simulink model "Par_model_sim_CHB5"  (R2023b)
settings: Solver=FixedStepAuto  StartTime=0.0  StopTime=5  FixedStep=1e-6  RelTol=1e-3
InitFcn:
  | sysinit
values from neighbouring files (symbols this model uses):
  C = 0.0234    [sysinit.m]
  f_out = frequency_out_start : frequency_out_interval : frequency_out_end    [simout_chb_par.m]    (also in simout_chbjt_par.m = frequency_modulate_start : frequency_modulate_interval : fre)
  f_switch = 250    [sysinit.m]
  fn = 50    [sysinit.m]
  L = 0.002    [sysinit.m]
  L_ori = 0.02    [sysinit.m]
  L_sec = 0.06    [sysinit.m]
  m_par = modulate_radio_start : modulate_radio_interval : modulate_radio_end    [simout_chb_par.m]
  P0 = 8e6    (= 8000000)    [sysinit.m]
  R = 1.5    [sysinit.m]
  Source_Amp = 10000    [sysinit.m]
  st = 1e-6    (= 1e-06)    [sysinit.m]
  Td = 15e-7    (= 1.5e-06)    [sysinit.m]
  Ul_in = 1900    [sysinit.m]
undefined symbols (not defined in the file or in its folder): D1, Delta
libraries: spsSeriesRLCBranchLib x63, spsDiodeLib x30, simulink x24, spsIGBTLib x24, spsCurrentMeasurementLib x10, spsThreePhaseVIMeasurementLib x7, spsOnDelayLib x6, spsUniversalBridgeLib x6, spsVoltageMeasurementLib x3, spsThreePhaseTransformerThreeWindingsLib x3, spsThreePhaseProgrammableVoltageSourceLib x1, spsGroundLib x1
(part 2 of 2)

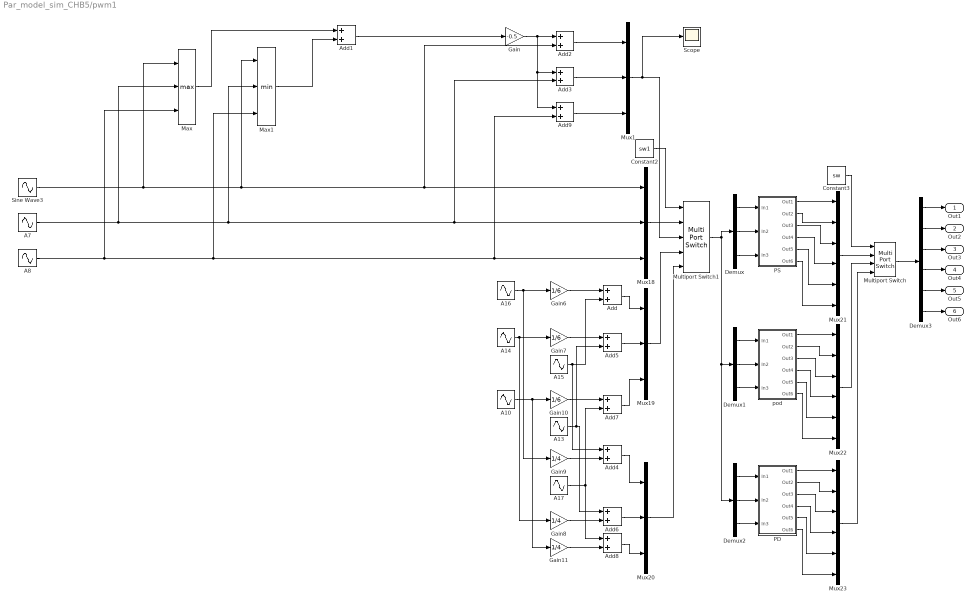
== system Par_model_sim_CHB5/pwm1 ==
  A10 : Sin  Amplitude=m*1000  Frequency=2*pi*f*3  Phase=pi+2*pi/3  SampleTime=0
  A13 : Sin  Amplitude=m*1000  Frequency=2*pi*f  Phase=pi-2*pi/3  SampleTime=0
  A14 : Sin  Amplitude=m*1000  Frequency=2*pi*f*3  Phase=pi-2*pi/3  SampleTime=0
  A15 : Sin  Amplitude=m*1000  Frequency=2*pi*f  Phase=pi  SampleTime=0
  A16 : Sin  Amplitude=m*1000  Frequency=2*pi*f*3  Phase=pi  SampleTime=0
  A17 : Sin  Amplitude=m*1000  Frequency=2*pi*f  Phase=pi+2*pi/3  SampleTime=0
  A7 : Sin  Amplitude=m*1000  Frequency=2*pi*f  Phase=-2*pi/3  SampleTime=0
  A8 : Sin  Amplitude=m*1000  Frequency=2*pi*f  Phase=2*pi/3  SampleTime=0
  Add{,1..9} (10 alike) : Sum
  Constant2 : Constant  Value=sw1
  Constant3 : Constant  Value=sw
  Demux : Demux  Outputs=3
  Demux1 : Demux  Outputs=3
  Demux2 : Demux  Outputs=3
  Demux3 : Demux  Outputs=6
  Gain : Gain  Gain=-0.5
  Gain10 : Gain  Gain=1/6
  Gain11 : Gain  Gain=1/4
  Gain6 : Gain  Gain=1/6
  Gain7 : Gain  Gain=1/6
  Gain8 : Gain  Gain=1/4
  Gain9 : Gain  Gain=1/4
  Max : MinMax  Function=max  Inputs=3
  Max1 : MinMax  Inputs=3
  Multiport Switch : MultiPortSwitch  SaturateOnIntegerOverflow=off  InputSameDT=off
  Multiport Switch1 : MultiPortSwitch  Inputs=4  SaturateOnIntegerOverflow=off  InputSameDT=off
  Mux{1,18..20} (4 alike) : Mux  Inputs=3
  Mux21 : Mux  Inputs=6
  Mux22 : Mux  Inputs=6
  Mux23 : Mux  Inputs=6
  PD : Subsystem
  PS : Subsystem
  Scope : Scope
  Sine Wave3 : Sin  Amplitude=m*1000  Frequency=2*pi*f  SampleTime=0
  pod : Subsystem
  Out1 : Outport
  Out2 : Outport  Port=2
  Out3 : Outport  Port=3
  Out4 : Outport  Port=4
  Out5 : Outport  Port=5
  Out6 : Outport  Port=6
  wires:
  Gain8/1 -> Add6/2
  Demux3/2 -> Out2/1
  Demux1/1 -> pod/1(In1)
  Mux19/1 -> Multiport Switch1/4
  Demux3/6 -> Out6/1
  A10/1 -> Gain11/1, Gain10/1
  PD/1(Out1) -> Mux23/1
  PD/3(Out3) -> Mux23/3
  PD/2(Out2) -> Mux23/2
  Demux3/5 -> Out5/1
  PD/4(Out4) -> Mux23/4
  A13/1 -> Add5/2, Add6/1
  Demux2/1 -> PD/1(In1)
  Demux2/3 -> PD/3(In3)
  PD/5(Out5) -> Mux23/5
  PD/6(Out6) -> Mux23/6
  Add8/1 -> Mux20/3
  Add7/1 -> Mux19/3
  Add5/1 -> Mux19/2
  Add6/1 -> Mux20/2
  Constant2/1 -> Multiport Switch1/1
  PS/3(Out3) -> Mux21/3
  PS/4(Out4) -> Mux21/4
  PS/5(Out5) -> Mux21/5
  PS/2(Out2) -> Mux21/2
  Constant3/1 -> Multiport Switch/1
  Mux20/1 -> Multiport Switch1/5
  Gain10/1 -> Add7/1
  Gain7/1 -> Add5/1
  Mux21/1 -> Multiport Switch/2
  A8/1 -> Max/3, Max1/3, Add9/2, Mux18/3
  Gain9/1 -> Add4/2
  Gain6/1 -> Add/1
  Gain11/1 -> Add8/2
  Demux1/3 -> pod/3(In3)
  Demux1/2 -> pod/2(In2)
  Demux/3 -> PS/3(In3)
  Demux3/3 -> Out3/1
  Sine Wave3/1 -> Max/1, Max1/1, Add2/2, Mux18/1
  pod/4(Out4) -> Mux22/4
  pod/1(Out1) -> Mux22/1
  pod/3(Out3) -> Mux22/3
  pod/2(Out2) -> Mux22/2
  Demux3/4 -> Out4/1
  Multiport Switch/1 -> Demux3/1
  Demux2/2 -> PD/2(In2)
  Demux/1 -> PS/1(In1)
  Demux/2 -> PS/2(In2)
  pod/6(Out6) -> Mux22/6
  pod/5(Out5) -> Mux22/5
  PS/6(Out6) -> Mux21/6
  Demux3/1 -> Out1/1
  PS/1(Out1) -> Mux21/1
  Add/1 -> Mux19/1
  Add4/1 -> Mux20/1
  Multiport Switch1/1 -> Demux/1, Demux1/1, Demux2/1
  Mux18/1 -> Multiport Switch1/2
  Mux22/1 -> Multiport Switch/3
  Mux23/1 -> Multiport Switch/4
  A17/1 -> Add8/1, Add7/2
  A16/1 -> Gain9/1, Gain6/1
  A15/1 -> Add4/1, Add/2
  A14/1 -> Gain7/1, Gain8/1
  Max/1 -> Add1/1
  Max1/1 -> Add1/2
  Add1/1 -> Gain/1
  Gain/1 -> Add9/1, Add3/1, Add2/1
  Add9/1 -> Mux1/3
  Add3/1 -> Mux1/2
  Add2/1 -> Mux1/1
  A7/1 -> Max/2, Max1/2, Add3/2, Mux18/2
  Mux1/1 -> Scope/1, Multiport Switch1/3

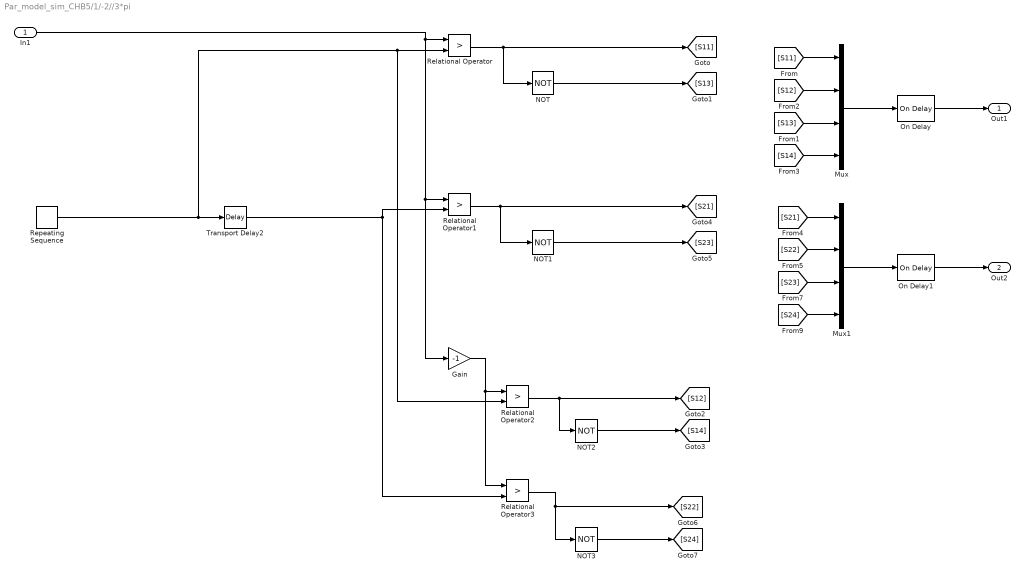
== system Par_model_sim_CHB5/1/-2//3*pi ==
  In1 : Inport
  Gain : Gain  Gain=-1
  Mux : Mux
  Mux1 : Mux
  NOT{,1..3} (4 alike) : Logic  Operator=NOT  AllPortsSameDT=off  OutDataTypeStr=boolean
  On Delay : spsOnDelayLib/On Delay  DelayType=On delay  delay=ttd  ic=0  Ts=0
  On Delay1 : spsOnDelayLib/On Delay  DelayType=On delay  delay=ttd  ic=0  Ts=0
  Relational Operator{,1..3} (4 alike) : RelationalOperator  Operator=>  OutDataTypeStr=boolean  RndMeth=Simplest  InputSameDT=off
  Repeating Sequence : simulink/Sources/Repeating Sequence  rep_seq_t=[0 0.5 1]/f_car  rep_seq_y=[-1 1 -1]*1000
  Transport Delay2 : TransportDelay  DelayTime=tt/f_car  BufferSize=3072
  Out1 : Outport
  Out2 : Outport  Port=2
  wires:
  On Delay1/1 -> Out2/1
  On Delay/1 -> Out1/1
  NOT/1 -> [S13]
  Transport Delay2/1 -> Relational Operator1/2, Relational Operator3/2
  [S14] -> Mux/4
  [S23] -> Mux1/3
  [S12] -> Mux/2
  In1/1 -> Gain/1, Relational Operator1/1, Relational Operator/1
  NOT2/1 -> [S14]
  [S21] -> Mux1/1
  Relational Operator1/1 -> NOT1/1, [S21]
  [S22] -> Mux1/2
  NOT3/1 -> [S24]
  Mux/1 -> On Delay/1
  Repeating Sequence/1 -> Relational Operator2/2, Relational Operator/2, Transport Delay2/1
  [S24] -> Mux1/4
  Gain/1 -> Relational Operator3/1, Relational Operator2/1
  [S13] -> Mux/3
  Relational Operator2/1 -> NOT2/1, [S12]
  [S11] -> Mux/1
  Relational Operator/1 -> NOT/1, [S11]
  NOT1/1 -> [S23]
  Mux1/1 -> On Delay1/1
  Relational Operator3/1 -> [S22], NOT3/1

== system Par_model_sim_CHB5/1/0 ==
  In1 : Inport
  Gain : Gain  Gain=-1
  Mux : Mux
  Mux1 : Mux
  NOT{,1..3} (4 alike) : Logic  Operator=NOT  AllPortsSameDT=off  OutDataTypeStr=boolean
  On Delay1 : spsOnDelayLib/On Delay  DelayType=On delay  delay=ttd  ic=0  Ts=0
  On Delay2 : spsOnDelayLib/On Delay  DelayType=On delay  delay=ttd  ic=0  Ts=0
  Relational Operator{,1..3} (4 alike) : RelationalOperator  Operator=>  OutDataTypeStr=boolean  RndMeth=Simplest  InputSameDT=off
  Repeating Sequence : simulink/Sources/Repeating Sequence  rep_seq_t=[0 0.5 1]/f_car  rep_seq_y=[-1 1 -1]*1000
  Transport Delay2 : TransportDelay  DelayTime=tt/f_car  BufferSize=3072
  Out1 : Outport
  Out2 : Outport  Port=2
  wires:
  On Delay2/1 -> Out1/1
  On Delay1/1 -> Out2/1
  Relational Operator3/1 -> NOT3/1, [S22]
  Mux1/1 -> On Delay1/1
  NOT1/1 -> [S23]
  Relational Operator/1 -> [S11], NOT/1
  [S11] -> Mux/1
  Relational Operator2/1 -> [S12], NOT2/1
  [S13] -> Mux/3
  Gain/1 -> Relational Operator2/1, Relational Operator3/1
  [S24] -> Mux1/4
  Repeating Sequence/1 -> Transport Delay2/1, Relational Operator/2, Relational Operator2/2
  Mux/1 -> On Delay2/1
  NOT3/1 -> [S24]
  [S22] -> Mux1/2
  Relational Operator1/1 -> [S21], NOT1/1
  [S21] -> Mux1/1
  NOT2/1 -> [S14]
  In1/1 -> Relational Operator/1, Relational Operator1/1, Gain/1
  [S12] -> Mux/2
  [S23] -> Mux1/3
  [S14] -> Mux/4
  Transport Delay2/1 -> Relational Operator3/2, Relational Operator1/2
  NOT/1 -> [S13]

== system Par_model_sim_CHB5/1/2//3*pi ==
  In1 : Inport
  Gain : Gain  Gain=-1
  Mux : Mux
  Mux1 : Mux
  NOT{,1..3} (4 alike) : Logic  Operator=NOT  AllPortsSameDT=off  OutDataTypeStr=boolean
  On Delay : spsOnDelayLib/On Delay  DelayType=On delay  delay=ttd  ic=0  Ts=0
  On Delay1 : spsOnDelayLib/On Delay  DelayType=On delay  delay=ttd  ic=0  Ts=0
  Relational Operator{,1..3} (4 alike) : RelationalOperator  Operator=>  OutDataTypeStr=boolean  RndMeth=Simplest  InputSameDT=off
  Repeating Sequence : simulink/Sources/Repeating Sequence  rep_seq_t=[0 0.5 1]/f_car  rep_seq_y=[-1 1 -1]*1000
  Transport Delay2 : TransportDelay  DelayTime=tt/f_car  BufferSize=3072
  Out1 : Outport
  Out2 : Outport  Port=2
  wires:
  On Delay1/1 -> Out2/1
  On Delay/1 -> Out1/1
  Relational Operator3/1 -> NOT3/1, [S22]
  Mux1/1 -> On Delay1/1
  NOT1/1 -> [S23]
  Relational Operator/1 -> [S11], NOT/1
  [S11] -> Mux/1
  Relational Operator2/1 -> [S12], NOT2/1
  [S13] -> Mux/3
  Gain/1 -> Relational Operator2/1, Relational Operator3/1
  [S24] -> Mux1/4
  Repeating Sequence/1 -> Transport Delay2/1, Relational Operator/2, Relational Operator2/2
  Mux/1 -> On Delay/1
  NOT3/1 -> [S24]
  [S22] -> Mux1/2
  Relational Operator1/1 -> [S21], NOT1/1
  [S21] -> Mux1/1
  NOT2/1 -> [S14]
  In1/1 -> Relational Operator/1, Relational Operator1/1, Gain/1
  [S12] -> Mux/2
  [S23] -> Mux1/3
  [S14] -> Mux/4
  Transport Delay2/1 -> Relational Operator3/2, Relational Operator1/2
  NOT/1 -> [S13]

== system Par_model_sim_CHB5/1/Subsystem ==
  In1 : Inport
  In2 : Inport  Port=2
  In3 : Inport  Port=3
  Add{1..3,9} (4 alike) : Sum
  Gain : Gain  Gain=-0.5
  Max : MinMax  Function=max  Inputs=3
  Max1 : MinMax  Inputs=3
  Out1 : Outport
  Out2 : Outport  Port=2
  Out3 : Outport  Port=3
  wires:
  Add3/1 -> Out2/1
  Add2/1 -> Out1/1
  Add9/1 -> Out3/1
  Add1/1 -> Gain/1
  Max1/1 -> Add1/2
  Max/1 -> Add1/1
  Gain/1 -> Add2/1, Add3/1, Add9/1
  In1/1 -> Max/1, Add2/2, Max1/1
  In3/1 -> Max/3, Max1/3, Add9/2
  In2/1 -> Max/2, Max1/2, Add3/2

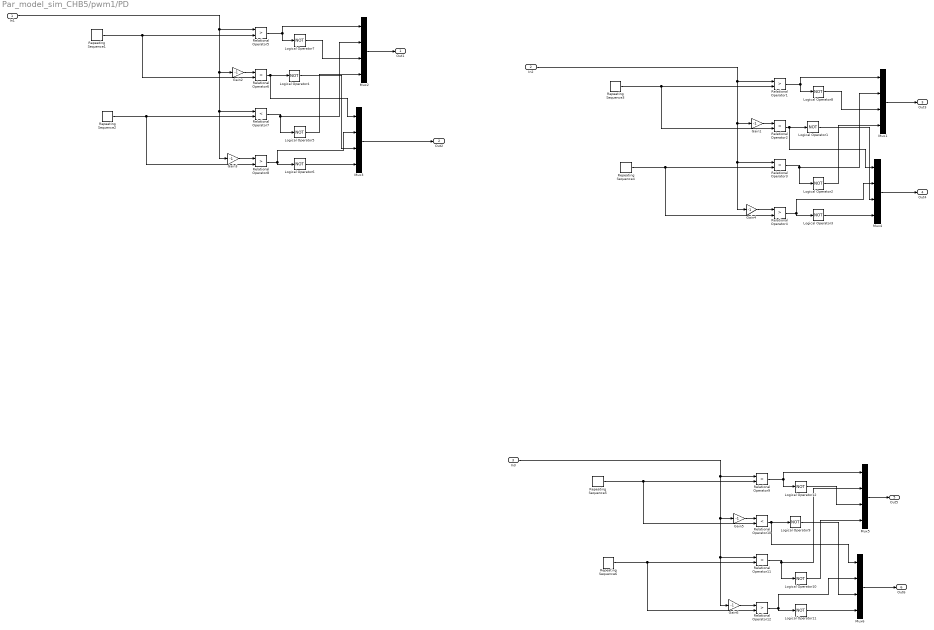
== system Par_model_sim_CHB5/pwm1/PD ==
  In1 : Inport
  In2 : Inport  Port=2
  In3 : Inport  Port=3
  Gain{1..6} (6 alike) : Gain  Gain=-1
  Logical Operator{1..12} (12 alike) : Logic  Operator=NOT  AllPortsSameDT=off  OutDataTypeStr=boolean
  Mux{1..6} (6 alike) : Mux
  Relational Operator{1,4..5,8..9,12} (6 alike) : RelationalOperator  Operator=>  OutDataTypeStr=boolean  RndMeth=Simplest  InputSameDT=off
  Relational Operator{2..3,6..7,10..11} (6 alike) : RelationalOperator  Operator=<  OutDataTypeStr=boolean  RndMeth=Simplest  InputSameDT=off
  Repeating Sequence1 : simulink/Sources/Repeating Sequence  rep_seq_t=[0 0.5 1]/f_carrier  rep_seq_y=[0 1 0]*1000
  Repeating Sequence2 : simulink/Sources/Repeating Sequence  rep_seq_t=[0 0.5 1]/f_carrier  rep_seq_y=[-1 0 -1]*1000
  Repeating Sequence3 : simulink/Sources/Repeating Sequence  rep_seq_t=[0 0.5 1]/f_carrier  rep_seq_y=[0 1 0]*1000
  Repeating Sequence4 : simulink/Sources/Repeating Sequence  rep_seq_t=[0 0.5 1]/f_carrier  rep_seq_y=[-1 0 -1]*1000
  Repeating Sequence5 : simulink/Sources/Repeating Sequence  rep_seq_t=[0 0.5 1]/f_carrier  rep_seq_y=[0 1 0]*1000
  Repeating Sequence6 : simulink/Sources/Repeating Sequence  rep_seq_t=[0 0.5 1]/f_carrier  rep_seq_y=[-1 0 -1]*1000
  Out1 : Outport
  Out2 : Outport  Port=2
  Out3 : Outport  Port=3
  Out4 : Outport  Port=4
  Out5 : Outport  Port=5
  Out6 : Outport  Port=6
  wires:
  Logical Operator4/1 -> Mux3/3
  In1/1 -> Gain3/1, Relational Operator7/1, Gain2/1, Relational Operator5/1
  Relational Operator5/1 -> Logical Operator7/1, Mux2/1
  Gain2/1 -> Relational Operator6/1
  Repeating Sequence1/1 -> Relational Operator6/2, Relational Operator5/2
  Logical Operator7/1 -> Mux2/3
  Logical Operator6/1 -> Mux3/4
  Relational Operator6/1 -> Mux3/1, Logical Operator4/1
  Repeating Sequence2/1 -> Relational Operator8/2, Relational Operator7/2
  Mux3/1 -> Out2/1
  Relational Operator7/1 -> Mux2/2, Logical Operator5/1
  Logical Operator5/1 -> Mux2/4
  Relational Operator8/1 -> Mux3/2, Logical Operator6/1
  Gain3/1 -> Relational Operator8/1
  Mux2/1 -> Out1/1
  Logical Operator1/1 -> Mux4/3
  In2/1 -> Gain4/1, Relational Operator3/1, Gain1/1, Relational Operator1/1
  Relational Operator1/1 -> Logical Operator8/1, Mux1/1
  Gain1/1 -> Relational Operator2/1
  Repeating Sequence3/1 -> Relational Operator2/2, Relational Operator1/2
  Logical Operator8/1 -> Mux1/3
  Logical Operator3/1 -> Mux4/4
  Relational Operator2/1 -> Mux4/1, Logical Operator1/1
  Repeating Sequence4/1 -> Relational Operator4/2, Relational Operator3/2
  Relational Operator3/1 -> Mux1/2, Logical Operator2/1
  Logical Operator2/1 -> Mux1/4
  Relational Operator4/1 -> Mux4/2, Logical Operator3/1
  Gain4/1 -> Relational Operator4/1
  Mux4/1 -> Out4/1
  Mux1/1 -> Out3/1
  Logical Operator9/1 -> Mux6/3
  In3/1 -> Gain6/1, Relational Operator11/1, Gain5/1, Relational Operator9/1
  Relational Operator9/1 -> Logical Operator12/1, Mux5/1
  Gain5/1 -> Relational Operator10/1
  Repeating Sequence5/1 -> Relational Operator10/2, Relational Operator9/2
  Logical Operator12/1 -> Mux5/3
  Logical Operator11/1 -> Mux6/4
  Relational Operator10/1 -> Mux6/1, Logical Operator9/1
  Repeating Sequence6/1 -> Relational Operator12/2, Relational Operator11/2
  Mux6/1 -> Out6/1
  Relational Operator11/1 -> Mux5/2, Logical Operator10/1
  Logical Operator10/1 -> Mux5/4
  Relational Operator12/1 -> Mux6/2, Logical Operator11/1
  Gain6/1 -> Relational Operator12/1
  Mux5/1 -> Out5/1

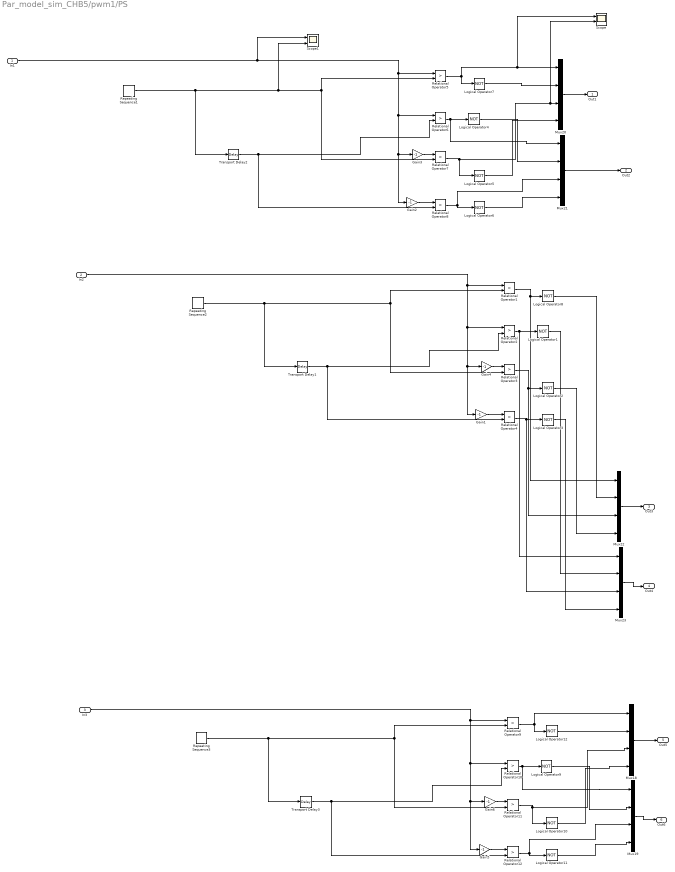
== system Par_model_sim_CHB5/pwm1/PS ==
  In1 : Inport
  In2 : Inport  Port=2
  In3 : Inport  Port=3
  Gain{1..6} (6 alike) : Gain  Gain=-1
  Logical Operator{1..12} (12 alike) : Logic  Operator=NOT  AllPortsSameDT=off  OutDataTypeStr=boolean
  Mux{18..23} (6 alike) : Mux
  Relational Operator{1..12} (12 alike) : RelationalOperator  Operator=>  OutDataTypeStr=boolean  RndMeth=Simplest  InputSameDT=off
  Repeating Sequence1 : simulink/Sources/Repeating Sequence  rep_seq_t=[0 0.5 1]/f_carrier  rep_seq_y=[-1 1 -1]*1000
  Repeating Sequence2 : simulink/Sources/Repeating Sequence  rep_seq_t=[0 0.5 1]/f_carrier  rep_seq_y=[-1 1 -1]*1000
  Repeating Sequence3 : simulink/Sources/Repeating Sequence  rep_seq_t=[0 0.5 1]/f_carrier  rep_seq_y=[-1 1 -1]*1000
  Scope : Scope  NumInputPorts=2
  Scope1 : Scope  NumInputPorts=2
  Transport Delay1 : TransportDelay  DelayTime=0.25*(1/f_carrier)  BufferSize=3072
  Transport Delay2 : TransportDelay  DelayTime=0.25*(1/f_carrier)  BufferSize=3072
  Transport Delay3 : TransportDelay  DelayTime=0.25*(1/f_carrier)  BufferSize=3072
  Out1 : Outport
  Out2 : Outport  Port=2
  Out3 : Outport  Port=3
  Out4 : Outport  Port=4
  Out5 : Outport  Port=5
  Out6 : Outport  Port=6
  wires:
  Mux22/1 -> Out3/1
  Mux18/1 -> Out5/1
  Mux23/1 -> Out4/1
  Mux20/1 -> Out1/1
  Mux19/1 -> Out6/1
  Mux21/1 -> Out2/1
  Logical Operator6/1 -> Mux21/4
  In1/1 -> Scope1/1, Relational Operator6/1, Gain2/1, Gain3/1, Relational Operator5/1
  Logical Operator7/1 -> Mux20/2
  Logical Operator5/1 -> Mux20/4
  Relational Operator7/1 -> Scope/2, Mux20/3, Logical Operator5/1
  Relational Operator8/1 -> Mux21/3, Logical Operator6/1
  Transport Delay2/1 -> Relational Operator8/2, Relational Operator6/2
  Gain3/1 -> Relational Operator7/1
  Relational Operator6/1 -> Mux21/1, Logical Operator4/1
  Logical Operator4/1 -> Mux21/2
  Gain2/1 -> Relational Operator8/1
  Repeating Sequence1/1 -> Transport Delay2/1, Scope1/2, Relational Operator7/2, Relational Operator5/2
  Relational Operator5/1 -> Scope/1, Mux20/1, Logical Operator7/1
  Logical Operator3/1 -> Mux23/4
  In2/1 -> Relational Operator2/1, Gain1/1, Gain4/1, Relational Operator1/1
  Relational Operator3/1 -> Mux22/3, Logical Operator2/1
  Gain4/1 -> Relational Operator3/1
  Transport Delay1/1 -> Relational Operator4/2, Relational Operator2/2
  Relational Operator4/1 -> Mux23/3, Logical Operator3/1
  Logical Operator8/1 -> Mux22/2
  Logical Operator2/1 -> Mux22/4
  Logical Operator1/1 -> Mux23/2
  Relational Operator2/1 -> Mux23/1, Logical Operator1/1
  Gain1/1 -> Relational Operator4/1
  Repeating Sequence2/1 -> Transport Delay1/1, Relational Operator3/2, Relational Operator1/2
  Relational Operator1/1 -> Mux22/1, Logical Operator8/1
  Logical Operator11/1 -> Mux19/4
  In3/1 -> Relational Operator10/1, Gain5/1, Gain6/1, Relational Operator9/1
  Relational Operator11/1 -> Mux18/3, Logical Operator10/1
  Gain6/1 -> Relational Operator11/1
  Transport Delay3/1 -> Relational Operator12/2, Relational Operator10/2
  Relational Operator12/1 -> Mux19/3, Logical Operator11/1
  Logical Operator12/1 -> Mux18/2
  Logical Operator10/1 -> Mux18/4
  Logical Operator9/1 -> Mux19/2
  Relational Operator10/1 -> Mux19/1, Logical Operator9/1
  Gain5/1 -> Relational Operator12/1
  Repeating Sequence3/1 -> Transport Delay3/1, Relational Operator11/2, Relational Operator9/2
  Relational Operator9/1 -> Mux18/1, Logical Operator12/1

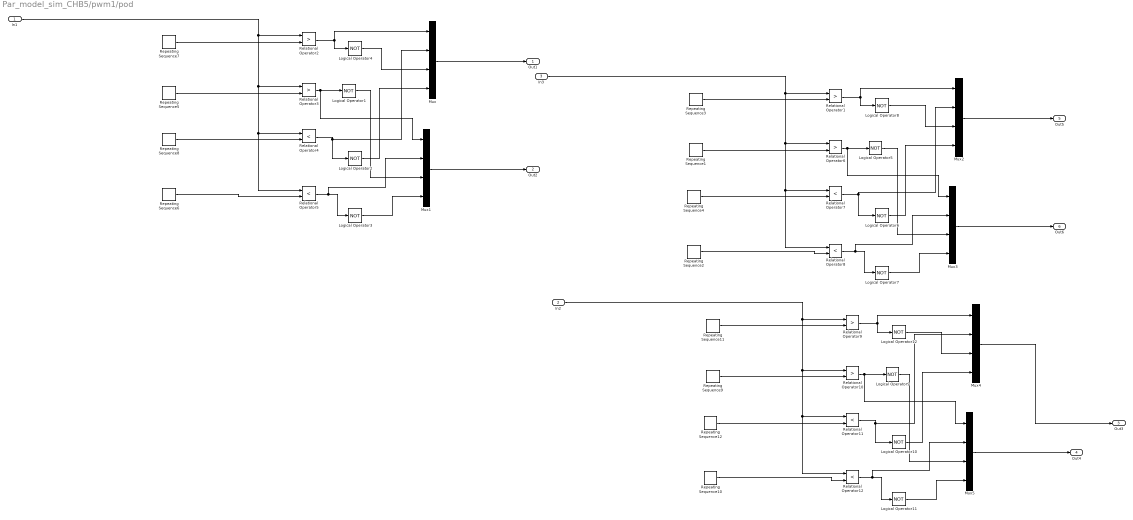
== system Par_model_sim_CHB5/pwm1/pod ==
  In1 : Inport
  In2 : Inport  Port=2
  In3 : Inport  Port=3
  Logical Operator{1..12} (12 alike) : Logic  Operator=NOT  AllPortsSameDT=off  OutDataTypeStr=boolean
  Mux{,1..5} (6 alike) : Mux
  Relational Operator{1..3,6,9..10} (6 alike) : RelationalOperator  Operator=>  OutDataTypeStr=boolean  RndMeth=Simplest  InputSameDT=off
  Relational Operator{4..5,7..8,11..12} (6 alike) : RelationalOperator  Operator=<  OutDataTypeStr=boolean  RndMeth=Simplest  InputSameDT=off
  Repeating Sequence1 : simulink/Sources/Repeating Sequence  rep_seq_t=[0 0.5 1]*(1/f_carrier)  rep_seq_y=[0 1 0]*500
  Repeating Sequence10 : simulink/Sources/Repeating Sequence  rep_seq_t=[0 0.5 1]*(1/f_carrier)  rep_seq_y=[-2 -1 -2]*500
  Repeating Sequence11 : simulink/Sources/Repeating Sequence  rep_seq_t=[0 0.5 1]*(1/f_carrier)  rep_seq_y=[1 2 1]*500
  Repeating Sequence12 : simulink/Sources/Repeating Sequence  rep_seq_t=[0 0.5 1]*(1/f_carrier)  rep_seq_y=[-1 0 -1]*500
  Repeating Sequence2 : simulink/Sources/Repeating Sequence  rep_seq_t=[0 0.5 1]*(1/f_carrier)  rep_seq_y=[-2 -1 -2]*500
  Repeating Sequence3 : simulink/Sources/Repeating Sequence  rep_seq_t=[0 0.5 1]*(1/f_carrier)  rep_seq_y=[1 2 1]*500
  Repeating Sequence4 : simulink/Sources/Repeating Sequence  rep_seq_t=[0 0.5 1]*(1/f_carrier)  rep_seq_y=[-1 0 -1]*500
  Repeating Sequence5 : simulink/Sources/Repeating Sequence  rep_seq_t=[0 0.5 1]*(1/f_carrier)  rep_seq_y=[0 1 0]*500
  Repeating Sequence6 : simulink/Sources/Repeating Sequence  rep_seq_t=[0 0.5 1]*(1/f_carrier)  rep_seq_y=[-2 -1 -2]*500
  Repeating Sequence7 : simulink/Sources/Repeating Sequence  rep_seq_t=[0 0.5 1]*(1/f_carrier)  rep_seq_y=[1 2 1]*500
  Repeating Sequence8 : simulink/Sources/Repeating Sequence  rep_seq_t=[0 0.5 1]*(1/f_carrier)  rep_seq_y=[-1 0 -1]*500
  Repeating Sequence9 : simulink/Sources/Repeating Sequence  rep_seq_t=[0 0.5 1]*(1/f_carrier)  rep_seq_y=[0 1 0]*500
  Out1 : Outport
  Out2 : Outport  Port=2
  Out3 : Outport  Port=3
  Out4 : Outport  Port=4
  Out5 : Outport  Port=5
  Out6 : Outport  Port=6
  wires:
  Relational Operator3/1 -> Mux1/1, Logical Operator1/1
  Relational Operator5/1 -> Mux1/2, Logical Operator3/1
  Relational Operator4/1 -> Mux/2, Logical Operator2/1
  Mux1/1 -> Out2/1
  Logical Operator4/1 -> Mux/3
  Repeating Sequence7/1 -> Relational Operator2/2
  Logical Operator2/1 -> Mux/4
  Mux/1 -> Out1/1
  Relational Operator2/1 -> Logical Operator4/1, Mux/1
  Logical Operator3/1 -> Mux1/4
  In1/1 -> Relational Operator5/1, Relational Operator4/1, Relational Operator3/1, Relational Operator2/1
  Repeating Sequence5/1 -> Relational Operator3/2
  Logical Operator1/1 -> Mux1/3
  Logical Operator5/1 -> Mux3/3
  Repeating Sequence1/1 -> Relational Operator6/2
  In3/1 -> Relational Operator1/1, Relational Operator6/1, Relational Operator7/1, Relational Operator8/1
  Logical Operator7/1 -> Mux3/4
  Relational Operator1/1 -> Mux2/1, Logical Operator8/1
  Mux2/1 -> Out5/1
  Logical Operator6/1 -> Mux2/4
  Repeating Sequence2/1 -> Relational Operator8/2
  Repeating Sequence3/1 -> Relational Operator1/2
  Logical Operator8/1 -> Mux2/3
  Mux3/1 -> Out6/1
  Relational Operator7/1 -> Logical Operator6/1, Mux2/2
  Relational Operator8/1 -> Mux3/2, Logical Operator7/1
  Repeating Sequence4/1 -> Relational Operator7/2
  Relational Operator6/1 -> Logical Operator5/1, Mux3/1
  Relational Operator10/1 -> Mux5/1, Logical Operator9/1
  Repeating Sequence12/1 -> Relational Operator11/2
  Relational Operator12/1 -> Mux5/2, Logical Operator11/1
  Relational Operator11/1 -> Mux4/2, Logical Operator10/1
  Mux5/1 -> Out4/1
  Logical Operator12/1 -> Mux4/3
  Repeating Sequence11/1 -> Relational Operator9/2
  Repeating Sequence10/1 -> Relational Operator12/2
  Logical Operator10/1 -> Mux4/4
  Mux4/1 -> Out3/1
  Relational Operator9/1 -> Logical Operator12/1, Mux4/1
  Logical Operator11/1 -> Mux5/4
  In2/1 -> Relational Operator12/1, Relational Operator11/1, Relational Operator10/1, Relational Operator9/1
  Repeating Sequence9/1 -> Relational Operator10/2
  Logical Operator9/1 -> Mux5/3
  Repeating Sequence8/1 -> Relational Operator4/2
  Repeating Sequence6/1 -> Relational Operator5/2
